simulink model "gm_RNN_Activation"  (R2020b)
settings: Solver=VariableStepAuto  StartTime=0.0  StopTime=10.0  RelTol=1e-3
libraries: hdlmdlgenlib x1
settings Model: Creator=chank  LastModifiedBy=chank
settings OptimizationCC: BlockReduction=off  ConditionallyExecuteInputs=off
settings DebuggingCC: InheritedTsInSrcMsg=none

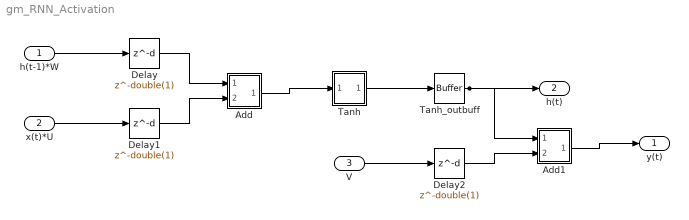
== system gm_RNN_Activation ==
  h(t-1)*W : Inport  OutDataTypeStr=single  PortDimensions=1  SampleTime=0.2
  x(t)*U : Inport  Port=2  OutDataTypeStr=single  PortDimensions=1  SampleTime=0.2
  V : Inport  Port=3  OutDataTypeStr=single  PortDimensions=1  SampleTime=0.2
  Add : Subsystem
      mask Display: disp('NFP\nadd');
  Add1 : Subsystem
      mask Display: disp('NFP\nadd');
  Delay : Delay  DelayLength=double(1)  InitialCondition=0  SampleTime=0.2
  Delay1 : Delay  DelayLength=double(1)  InitialCondition=0  SampleTime=0.2
  Delay2 : Delay  DelayLength=double(1)  InitialCondition=0  SampleTime=0.2
  Tanh : Subsystem
      mask Display: disp('NFP\ntrig');
  Tanh_outbuff : hdlmdlgenlib/Buffer
      settings: SourceProductBaseCode=SL
  y(t) : Outport
  h(t) : Outport  Port=2
  wires:
  h(t-1)*W/1 -> Delay/1
  x(t)*U/1 -> Delay1/1
  V/1 -> Delay2/1
  Delay/1 -> Add/1(In1)
  Delay1/1 -> Add/2(In2)
  Delay2/1 -> Add1/2(In2)
  Tanh_outbuff/1 -> Add1/1(In1), h(t)/1
  Add/1(Out1) -> Tanh/1(In1)
  Add1/1(Out1) -> y(t)/1
  Tanh/1(Out1) -> Tanh_outbuff/1

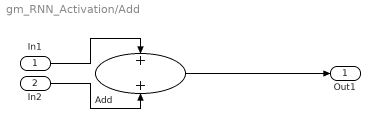
== system gm_RNN_Activation/Add ==
  In1 : Inport
  In2 : Inport  Port=2
  Add : Sum  OutDataTypeStr=single  SampleTime=0.2
  Out1 : Outport
  wires:
  In1/1 -> Add/1
  In2/1 -> Add/2
  Add/1 -> Out1/1

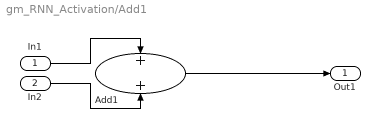
== system gm_RNN_Activation/Add1 ==
  In1 : Inport
  In2 : Inport  Port=2
  Add1 : Sum  OutDataTypeStr=single  SampleTime=0.2
  Out1 : Outport
  wires:
  In1/1 -> Add1/1
  In2/1 -> Add1/2
  Add1/1 -> Out1/1

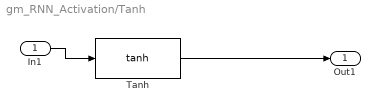
== system gm_RNN_Activation/Tanh ==
  In1 : Inport
  Tanh : Trigonometry  Operator=tanh  SampleTime=0.2
  Out1 : Outport
  wires:
  In1/1 -> Tanh/1
  Tanh/1 -> Out1/1
